simulink model "max_I_dutycycle"  (R2024b)
settings: Solver=VariableStepAuto  StartTime=0.0  StopTime=165e-3  RelTol=1e-3
libraries: eeGeneralControl x3, spsMosfetLib x2, simulink x2, spsCurrentMeasurementLib x1, spsDCVoltageSourceLib x1, spsDiodeLib x1, spsPVArrayLib x1, spsSeriesRLCBranchLib x1, spsVoltageMeasurementLib x1, sps_lib x1
settings Model: LastModifiedBy=deso

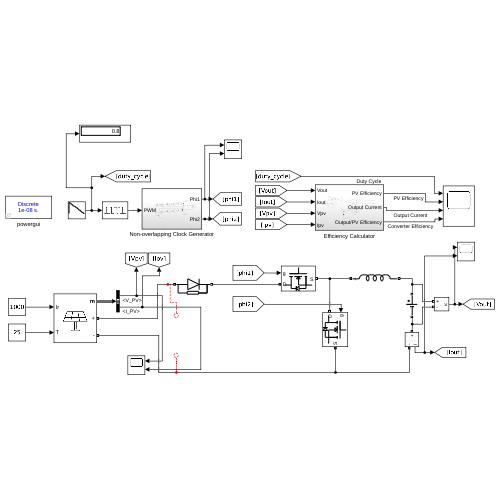
[thumbnail: Simulink's stored preview of the top-level diagram]
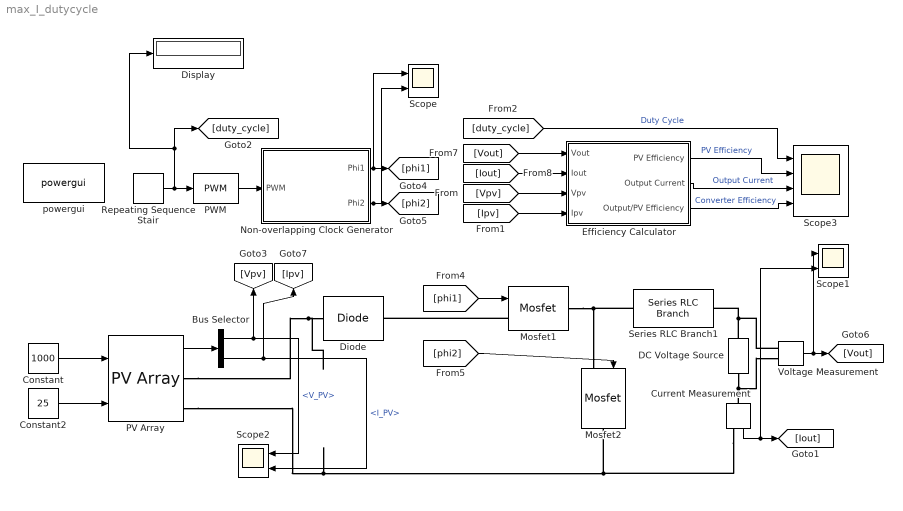
== system max_I_dutycycle ==
  Bus Selector : BusSelector  OutputSignals=V_PV,I_PV
  Constant : Constant  Value=1000
  Constant2 : Constant  Value=25
  Current Measurement : spsCurrentMeasurementLib/Current Measurement  PhasorSimulation=off  OutputType=Complex  PSBequivalent=0
  DC Voltage Source : spsDCVoltageSourceLib/DC Voltage Source  Amplitude=15  Measurements=None
  Diode : spsDiodeLib/Diode  Ron=1e-3  Lon=1e-9  Vf=0.7  IC=0  UseSnubber=0  Rs=500  Cs=500e-9  Measurements=off
  Display : Display
  Efficiency Calculator : Subsystem
  Mosfet1 : spsMosfetLib/Mosfet  Ron=10e-3  Lon=1e-9  Rd=0.01  Vfd=0.7  IC=0  Rs=1e5  Cs=inf  Measurements=off
  Mosfet2 : spsMosfetLib/Mosfet  Ron=10e-3  Lon=1e-9  Rd=0.01  Vfd=0.7  IC=0  Rs=1e5  Cs=inf  Measurements=off
  Non-overlapping Clock Generator : Subsystem
  PV Array : spsPVArrayLib/PV Array  Npar=1  Nser=1  PlotType=one module @ 25 deg.C & specified irradiances  S_vec="[ 1000  500  100 ]"  Temp_C_vec="[ 45 25  ]"  ModuleName=Ablytek 6MN6A280  PlotWhenSelected=off  Pm=280.0896  Ncell=60  Voc=39.31  Isc=9.51  Vm=31.26  Im=8.96  beta_Voc_pc=-0.3137  alpha_Isc_pc=0.052103  beta_Voc=-0.12331  alpha_Isc=0.004955  IL=9.5578  I0=5.7114e-11  nI=0.98731  Rsh=279.2025  Rs=0.39513  RobustModel=off  RobustCellTemperature=313.3991  BAL=on  Tc=1e-6  Tfilter=5e-5
  PWM : simulink/Discontinuities/PWM  DisableCoverage=on  Period=4e-5  InitialDelay=0  DisallowZeroDutyCycle=off  RunAtFixedTimeIntervals=off  SampleTime=0.1
  Repeating Sequence Stair : simulink/Sources/Repeating Sequence Stair  OutValues=[0.80 0.76 0.72 0.68 0.66 0.62 0.59 0.56 0.52 0.48 0.44]  tsamp=15e-3  OutMin=[]  OutMax=[]  OutDataTypeStr=double  OutputDataTypeScalingMode=double  OutDataType=fixdt(0,8)  ConRadixGroup=Best Precision: Vector-wise  OutScaling=2^-12
  Scope : Scope  NumInputPorts=2
  Scope1 : Scope  NumInputPorts=2
  Scope2 : Scope  NumInputPorts=2
  Scope3 : Scope  NumInputPorts=4
  Series RLC Branch1 : spsSeriesRLCBranchLib/Series RLC Branch  LConnTagsString=__new0  RConnTagsString=__new0  BranchType=L  Resistance=0  Inductance=10e-6  SetiL0=off  InitialCurrent=0  Capacitance=1000e-6  Setx0=off  InitialVoltage=0  Measurements=None
  Voltage Measurement : spsVoltageMeasurementLib/Voltage Measurement  PhasorSimulation=off  OutputType=Complex  PSBequivalent=0
  powergui : sps_lib/powergui  Priority=1  SimulationMode=Discrete  SampleTime=1e-8  frequency=60  Iterations=50  frequencyindice=0  Pbase=100e6  ErrMax=1e-4  UnitsV=kV  UnitsW=MW  buscounter=0  FunctionMessages=off  echomessages=off  EnableUseOfTLC=off  CurrentSourceSwitches=off  DisableSnubberDevices=off  DisableRonSwitches=off  DisableVfSwitches=off  DisplayEquations=off  AutomaticDiscreteSolvers=off  SolverType=Tustin/Backward Euler (TBE)  Interpol=off  ExternalGateDelay=off  methode=off  Ts=100  x0status=blocks  SPID=on  SwTol=0  HookPort=off  NonlinearTolerance=1e-4  nMaxIteration=100  ContinueOnMaxIteration=off  RestoreLinks=warning  ResistiveCurrentMeasurement=off  Frange=[0:2:500]  Ylog=off  Xlog=on  ShowGrid=off  save=off  variable=ZData  structure=0  ZoomFFT=off  StartTime=0.0  cycles=1  DisplayStyle=1  fundamental=60  FreqAxis=off  MaxFrequency=1000  frequencyindicesteady=1  RmsSteady=1  display=off
  wires:
  Constant2/1 -> PV Array/2
  PV Array/1 -> Bus Selector/1
  Constant/1 -> PV Array/1
  [phi2] -> Mosfet2/1
  [phi1] -> Mosfet1/1
  Voltage Measurement/1 -> Scope1/1, [Vout]
  [Vout] -> Efficiency Calculator/1(Vout)
  [Iout] -> Efficiency Calculator/2(Iout)
  Bus Selector/1 -> Scope2/1, [Vpv]  "<V_PV>"
  Bus Selector/2 -> Scope2/2, [Ipv]  "<I_PV>"
  [Vpv] -> Efficiency Calculator/3(Vpv)
  [Ipv] -> Efficiency Calculator/4(Ipv)
  Efficiency Calculator/1(PV Efficiency) -> Scope3/2  "PV Efficiency"
  Efficiency Calculator/2(Output Current) -> Scope3/3  "Output Current"
  Efficiency Calculator/3(Output/PV Efficiency) -> Scope3/4  "Converter Efficiency"
  Repeating Sequence Stair/1 -> Display/1, [duty_cycle], PWM/1
  PWM/1 -> Non-overlapping Clock Generator/1(PWM)
  Non-overlapping Clock Generator/1(Phi1) -> Scope/1, [phi1]
  Non-overlapping Clock Generator/2(Phi2) -> Scope/2, [phi2]
  Current Measurement/1 -> Scope1/2, [Iout]
  [duty_cycle] -> Scope3/1  "Duty Cycle"
  connections:
  PV Array/RConn2 -- Current Measurement/RConn1 -- Mosfet2/RConn1
  Mosfet1/LConn1 -- Diode/RConn1
  Mosfet1/RConn1 -- Series RLC Branch1/LConn1 -- Mosfet2/LConn1
  PV Array/RConn1 -- Diode/LConn1
  Voltage Measurement/LConn1 -- Series RLC Branch1/RConn1 -- DC Voltage Source/RConn1
  DC Voltage Source/LConn1 -- Voltage Measurement/LConn2 -- Current Measurement/LConn1

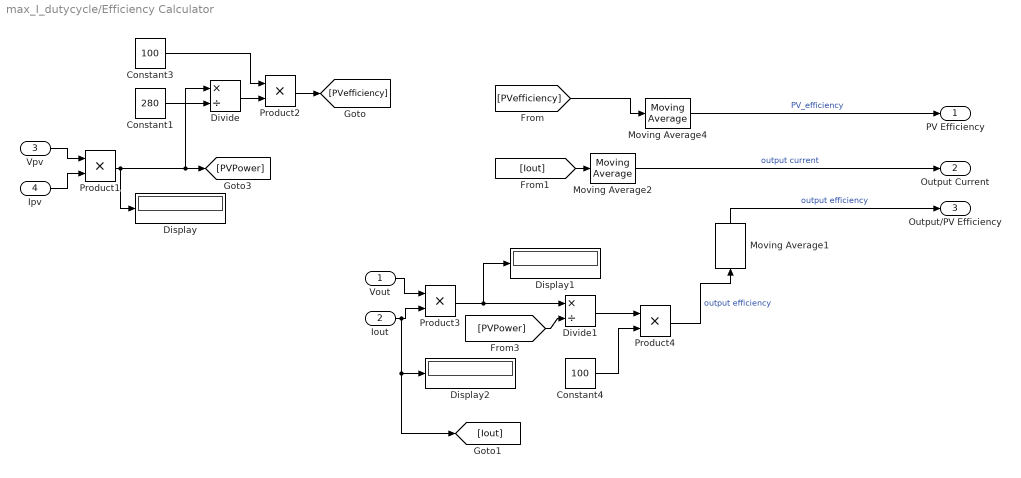
== system max_I_dutycycle/Efficiency Calculator ==
  Vout : Inport
  Iout : Inport  Port=2
  Vpv : Inport  Port=3
  Ipv : Inport  Port=4
  Constant1 : Constant  Value=280
  Constant3 : Constant  Value=100
  Constant4 : Constant  Value=100
  Display : Display
      settings: Format=decimal (Stored Integer)
  Display1 : Display
      settings: Format=decimal (Stored Integer)
  Display2 : Display
      settings: Format=decimal (Stored Integer)
  Divide : Product  Inputs=*/
  Divide1 : Product  Inputs=*/
  Moving Average1 : eeGeneralControl/Moving Average  VariantControl=Variant1  LabelModeActiveChoice=Discrete  f=25e3  x0=0  BufferSize=8192  Ts=1e-6
      settings: LibrarySourceBlock=ee_sl_lib/General Control/Moving Average
  Moving Average2 : eeGeneralControl/Moving Average  VariantControl=Variant1  LabelModeActiveChoice=Discrete  f=25e3  x0=0  BufferSize=8192  Ts=1e-6
      settings: LibrarySourceBlock=ee_sl_lib/General Control/Moving Average
  Moving Average4 : eeGeneralControl/Moving Average  VariantControl=Variant1  LabelModeActiveChoice=Discrete  f=25e3  x0=0  BufferSize=8192  Ts=1e-6
      settings: LibrarySourceBlock=ee_sl_lib/General Control/Moving Average
  Product{1..4} (4 alike) : Product
  PV Efficiency : Outport
  Output Current : Outport  Port=2
  Output/PV Efficiency : Outport  Port=3
  wires:
  Constant4/1 -> Product4/2
  [PVefficiency] -> Moving Average4/1
  Iout/1 -> [Iout], Display2/1, Product3/2
  Vout/1 -> Product3/1
  Divide1/1 -> Product4/1
  Product3/1 -> Display1/1, Divide1/1
  Moving Average1/1 -> Output/PV Efficiency/1  "output efficiency"
  Moving Average2/1 -> Output Current/1  "output current"
  Product4/1 -> Moving Average1/1  "output efficiency"
  [PVPower] -> Divide1/2
  [Iout] -> Moving Average2/1
  Moving Average4/1 -> PV Efficiency/1  "PV_efficiency"
  Divide/1 -> Product2/2
  Constant3/1 -> Product2/1
  Product1/1 -> Divide/1, [PVPower], Display/1
  Constant1/1 -> Divide/2
  Product2/1 -> [PVefficiency]
  Vpv/1 -> Product1/1
  Ipv/1 -> Product1/2

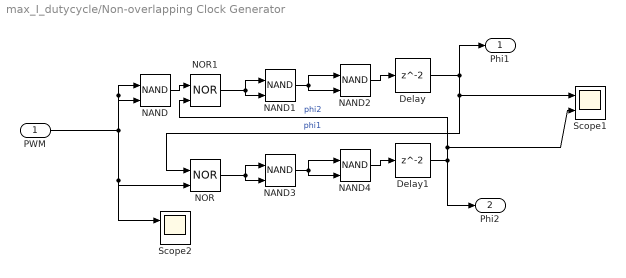
== system max_I_dutycycle/Non-overlapping Clock Generator ==
  PWM : Inport
  Delay : Delay  SampleTime=1e-6
  Delay1 : Delay  SampleTime=1e-6
  NAND{,1..4} (5 alike) : Logic  Operator=NAND  IconShape=distinctive  AllPortsSameDT=off  OutDataTypeStr=boolean
  NOR : Logic  Operator=NOR  IconShape=distinctive  AllPortsSameDT=off  OutDataTypeStr=boolean
  NOR1 : Logic  Operator=NOR  IconShape=distinctive  AllPortsSameDT=off  OutDataTypeStr=boolean
  Scope1 : Scope  NumInputPorts=2
  Scope2 : Scope  NumInputPorts=2
  Phi1 : Outport
  Phi2 : Outport  Port=2
  wires:
  NOR/1 -> NAND3/1, NAND3/2
  NAND3/1 -> NAND4/1, NAND4/2
  NAND/1 -> NOR1/1
  NOR1/1 -> NAND1/1, NAND1/2
  Delay1/1 -> NOR1/2, Scope1/2, Phi2/1  "phi2"
  NAND4/1 -> Delay1/1
  NAND2/1 -> Delay/1
  Delay/1 -> NOR/1, Scope1/1, Phi1/1  "phi1"
  NAND1/1 -> NAND2/1, NAND2/2
  PWM/1 -> Scope2/1, NOR/2, NAND/2, NAND/1
